simulink model "modelZSB"  (Simulink 8.3)
settings: Solver=ode4  StartTime=0.0  StopTime=0.2  FixedStep=0.01  RelTol=1e-3
settings Model: Creator=Chan Hwaiwing  LastModifiedBy=shubo
settings DataIOCC: SignalLoggingSaveFormat=Dataset
settings DebuggingCC: UnderspecifiedInitializationDetection=Simplified  MergeDetectMultiDrivingBlocksExec=error  FrameProcessingCompatibilityMsg=error  StateNameClashWarn=none
settings GRTTargetCC: CombineOutputUpdateFcns=on  GRTInterface=off
settings ConfigComp: CovCompData="CovMetricSettings\t  dw"  CovFilter=CovHTMLOptions  CovHtmlReporting=on  CovSaveCumulativeToWorkspaceVar=on  CovSaveSingleToWorkspaceVar=on  CovModelRefExcluded="CovExternalEMLEnable\t  off"  CovSFcnEnable=off

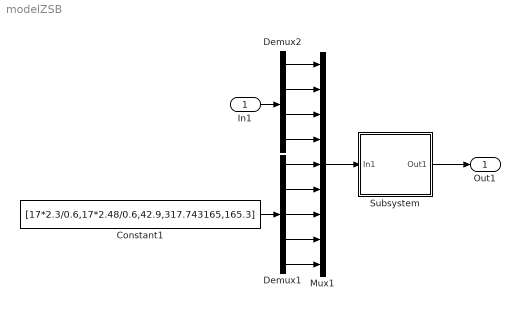
== system modelZSB ==
  In1 : Inport
  Constant1 : Constant  Value=[17*2.3/0.6,17*2.48/0.6,42.9,317.743165,165.3]
  Demux1 : Demux  Outputs=5
  Demux2 : Demux
  Mux1 : Mux  Inputs=9
  Subsystem : Subsystem
      mask help: Simulink:masks:GenSFuncDesc_MD
      mask Help: eval('feval(''rtwprivate'',''rtwhelpview'',''rtw_sfcn_block'')');
  Out1 : Outport
  wires:
  Subsystem/1(Out1) -> Out1/1
  Demux2/2 -> Mux1/2
  Demux2/4 -> Mux1/4
  Demux2/3 -> Mux1/3
  Demux2/1 -> Mux1/1
  Mux1/1 -> Subsystem/1(In1)
  In1/1 -> Demux2/1
  Constant1/1 -> Demux1/1
  Demux1/5 -> Mux1/9
  Demux1/2 -> Mux1/6
  Demux1/3 -> Mux1/7
  Demux1/4 -> Mux1/8
  Demux1/1 -> Mux1/5

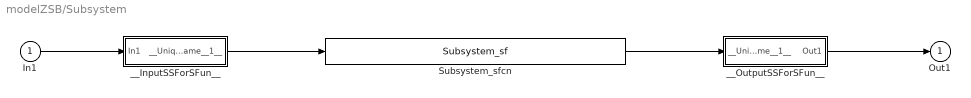
== system modelZSB/Subsystem ==
  In1 : Inport
  Subsystem_sfcn : S-Function  FunctionName=Subsystem_sf  SFunctionModules=""  EnableBusSupport=off  mask{rtw_sf_name=Subsystem_sf, showVar=off}
      mask prompts: rtw_sf_name "Simulink:masks:GenSFuncName_MP"; showVar "Simulink:masks:GenSFuncShowModuleList_MP"
      mask help: Simulink:masks:GenSFuncDesc_MD
      mask init:
      | displist = '';
      | if ~strcmp(get_param(gcb, 'FunctionName'), rtw_sf_name);
      |   set_param(gcb, 'FunctionName', rtw_sf_name);
      | end
      | % Check if we are generating code
      | rtw_mode = false;
      | if strcmpi(get_param(bdroot(gcb),'SimulationStatus'),'Initializing')
      | 	rtw_mode = strcmpi(get_param(bdroot(gcb),'BuildingRTWCode'),'on') && ...
      | 		~strcmpi(get_param(bdroot(gcb),'TargetStyle'),'SimulationTarget');
      | end
      | if showVar || rtw_mode
      | 	if exist('rtwsfunc') == 2 | exist('rtwsfunc') == 6
      | 		tmplist = rtwsfunc(rtw_sf_name,gcb);
      | 		tmplist = DAStudio.message('Simulink:masks:GenSFuncListOfModules_IC', tmplist);
      | 	elseif showVar
      | 		tmplist1 = DAStudio.message('Simulink:masks:GenSFuncListOfModules_IC', '');
      |         tmplist2 = DAStudio.message('Simulink:masks:GenSFuncNotLicensed_IC');
      |         tmplist = [tmplist1 tmplist2];
      |  	end
      | end
      | if showVar
      |   displist = tmplist;
      | end
      settings: CopyFcn=|
      | if ~strcmp(get_param(gcb,'Linkstatus'),'none') && ...
      | ~strcmp(get_param(gcb,'Linkstatus'),'implicit')
      |   set_param(gcb,'LinkStatus','none');
      | end
      mask Help: eval('feval(''rtwprivate'',''rtwhelpview'',''rtw_sfcn_block'')');
      mask Display:
      | port_label('input',1,'In1');
      | port_label('output',1,'Out1');
  __InputSSForSFun__ : Subsystem
  __OutputSSForSFun__ : Subsystem
  Out1 : Outport
  wires:
  In1/1 -> __InputSSForSFun__/1(In1)
  __InputSSForSFun__/1(__UniqueOutportName__1__) -> Subsystem_sfcn/1
  Subsystem_sfcn/1 -> __OutputSSForSFun__/1(__UniqueInportName__1__)
  __OutputSSForSFun__/1(Out1) -> Out1/1

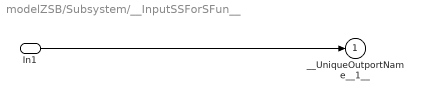
== system modelZSB/Subsystem/__InputSSForSFun__ ==
  In1 : Inport
  __UniqueOutportName__1__ : Outport
  wires:
  In1/1 -> __UniqueOutportName__1__/1

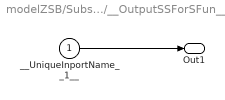
== system modelZSB/Subsystem/__OutputSSForSFun__ ==
  __UniqueInportName__1__ : Inport
  Out1 : Outport
  wires:
  __UniqueInportName__1__/1 -> Out1/1
